simulink model "Model_Simscape_V3"  (R2023a)
settings: Solver=VariableStepAuto  StartTime=0.0  StopTime=10.0  RelTol=1e-3
model workspace (MAT data in the model file):
  Air_density = 1.29
  Body_Temperature = 37
  CtrlData_Max = 100
  CtrlData_Min = 0
  Detpress_to_Vavle : object (value not decoded)
  E_respriatory = 10
  ExpValve : object (value not decoded)
  FRC = 2
  Fan : object (value not decoded)
  FanHousing : object (value not decoded)
  Flow_Resistance_1 : object (value not decoded)
  Flow_Resistance_2 : object (value not decoded)
  Hard_Stop : Lower_bound (value not decoded)
  InspValve : object (value not decoded)
  L_to_m3 = 0.001
  Mask : object (value not decoded)
  OxyValve : object (value not decoded)
  OxygenSensor : object (value not decoded)
  Pa_to_cmH2O = 0.0101974428892
  Percent_to_Unit = 0.01
  Pipe_1 : object (value not decoded)
  Pipe_2 : object (value not decoded)
  Pipe_3 : object (value not decoded)
  R_respiratory = 2
  Reservoir : Cross_area (value not decoded)
  Trachea : object (value not decoded)
  Volume_Max = 0.9
  cmH2O_to_Pa = 98.0638
  cmH2O_to_kPa = 0.0981
  lung : object (value not decoded)
  percentage_to_rpm = 600
values from neighbouring files (symbols this model uses):
  MIN_TO_S = 60.0    [MVEPP_DataDict.sldd]
  TO_HUNDRED = 0.01    [MVEPP_DataDict.sldd]
  TO_MILLI = 1000.0    [MVEPP_DataDict.sldd]
symbols that are objects in the model workspace (value not decoded): FanHousing, Flow_Resistance_1, Flow_Resistance_2, InspValve, lung, OxygenSensor
libraries: fl_lib x83, nesl_utility x17, SimscapeFluids_lib x4, aerolibatmos2 x1
(part 3 of 4)

== system Model_Simscape_V3/Subsystem/DiverPressSensor ==
  Data Type Conversion5 : DataTypeConversion  OutDataTypeStr=single  SaturateOnIntegerOverflow=off  RndMeth=Floor
  PS-Simulink Converter : nesl_utility/PS-Simulink Converter  PhysicalDomain=network_engine_domain  SubClassName=ps_output  LeftPortType=input  RightPortType=output  PseudoPeriodic=off  Frequencies=[]  VectorFormat=inherit  Unit=Pa  AffineConversion=off
  Pressure & Temperature Sensor (G) : fl_lib/Gas/Sensors/Pressure & Temperature Sensor (G)  reference=foundation.enum.MeasurementReference.difference  pressure=true  pressure_spec=foundation.enum.PressureMeasementSpec.Absolute  temperature=false
      settings: InternalSimscapePortConfiguration="{\"Bottom\":[],\"Left\":[{\"id\":\"A\",\"label\":\"A\",\"type\":\"foundation.gas.gas\"}],\"Right\":[{\"id\":\"B\",\"label\":\"B\",\"type\":\"foundation.gas.gas\"},{\"id\":\"P\",\"label\":\"P\",\"type\":\"output\"}],\"Top\":[]}"
  Reservoir (G)1 : fl_lib/Gas/Elements/Reservoir (G)  pressure_spec=foundation.enum.pressure_spec.atmospheric  reservoir_pressure=0.101325 MPa  reservoir_temperature=293.15 K  area_A=Reservoir.Cross_area m^2
  Unit Conversion : UnitConversion
  A : PMIOPort  Side=Left
  Press : Outport  Unit=hPa
  wires:
  PS-Simulink Converter/1 -> Unit Conversion/1
  Unit Conversion/1 -> Data Type Conversion5/1
  Data Type Conversion5/1 -> Press/1
  connections:
  Reservoir (G)1/LConn1 -- Pressure & Temperature Sensor (G)/RConn1
  Pressure & Temperature Sensor (G)/LConn1 -- A/RConn1
  Pressure & Temperature Sensor (G)/RConn2 -- PS-Simulink Converter/LConn1

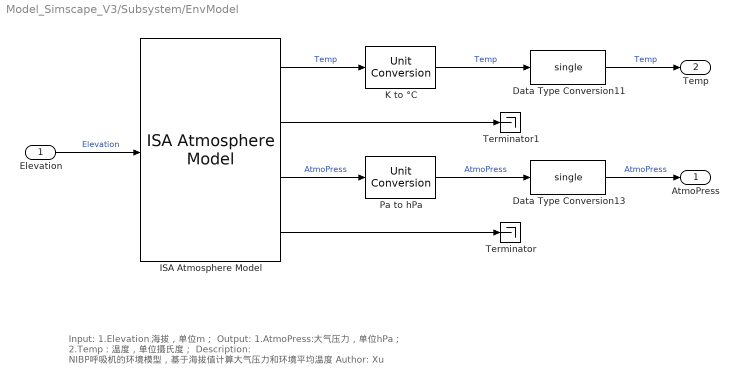
== system Model_Simscape_V3/Subsystem/EnvModel ==
  note: Input:
      | 	1.Elevation:海拔，单位m；
      | Output:
      | 	1.AtmoPress:大气压力，单位hPa；
      | 	2.Temp：温度，单位摄氏度；
      | Description:
      | 	NIBP呼吸机的环境模型，基于海拔值计算大气压力和环境平均温度
      | Author:
      | 	Xu
  Elevation : Inport  OutDataTypeStr=int16  Unit=m
  Data Type Conversion11 : DataTypeConversion  OutDataTypeStr=single  SaturateOnIntegerOverflow=off  RndMeth=Floor
  Data Type Conversion13 : DataTypeConversion  OutDataTypeStr=single  SaturateOnIntegerOverflow=off  RndMeth=Floor
  ISA Atmosphere Model : aerolibatmos2/ISA Atmosphere Model  custom=off  g=9.80665  gamma=1.4  R=287.0531  L=0.0065  h_trop=11000  h_strat=20000  rho0=1.225  P0=101325  T0=288.15  h0=0
  K to °C : UnitConversion  OutputType=Inherit: Inherit via back propagation
  Pa to hPa : UnitConversion  OutputType=Inherit: Inherit via back propagation
  Terminator : Terminator
  Terminator1 : Terminator
  AtmoPress : Outport  OutDataTypeStr=single  Unit=hPa
  Temp : Outport  Port=2  OutDataTypeStr=single  Unit=°C
  wires:
  Elevation/1 -> ISA Atmosphere Model/1  "Elevation"
  Pa to hPa/1 -> Data Type Conversion13/1  "AtmoPress"
  ISA Atmosphere Model/4 -> Terminator/1
  K to °C/1 -> Data Type Conversion11/1  "Temp"
  ISA Atmosphere Model/2 -> Terminator1/1
  ISA Atmosphere Model/3 -> Pa to hPa/1  "AtmoPress"
  ISA Atmosphere Model/1 -> K to °C/1  "Temp"
  Data Type Conversion11/1 -> Temp/1  "Temp"
  Data Type Conversion13/1 -> AtmoPress/1  "AtmoPress"

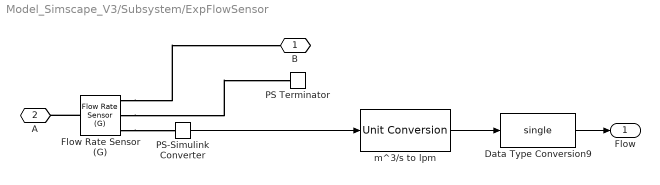
== system Model_Simscape_V3/Subsystem/ExpFlowSensor ==
  Data Type Conversion9 : DataTypeConversion  OutDataTypeStr=single  SaturateOnIntegerOverflow=off  RndMeth=Floor
  Flow Rate Sensor (G) : fl_lib/Gas/Sensors/Flow Rate Sensor (G)  mass_flow_measure=true  volumetric_flow_measure=true  volumetric_flow_conditions=foundation.enum.volumetric_flow_conditions.actual  p_std=0.101325 MPa  T_std=20 degC  energy_flow_measure=false
      settings: InternalSimscapePortConfiguration="{\"Bottom\":[],\"Left\":[{\"id\":\"A\",\"label\":\"A\",\"type\":\"foundation.gas.gas\"}],\"Right\":[{\"id\":\"B\",\"label\":\"B\",\"type\":\"foundation.gas.gas\"},{\"id\":\"M\",\"label\":\"M\",\"type\":\"output\"},{\"id\":\"V\",\"label\":\"V\",\"type\":\"output\"}],\"Top\":[]}"
  PS Terminator : fl_lib/Physical Signals/Sinks/PS Terminator
  PS-Simulink Converter : nesl_utility/PS-Simulink Converter  PhysicalDomain=network_engine_domain  SubClassName=ps_output  LeftPortType=input  RightPortType=output  PseudoPeriodic=off  Frequencies=[]  VectorFormat=inherit  Unit=m^3/s  AffineConversion=off
  m^3/s to lpm : UnitConversion
  B : PMIOPort  Side=Left
  A : PMIOPort  Port=2  Side=Right
  Flow : Outport  Unit=lpm
  wires:
  PS-Simulink Converter/1 -> m^3/s to lpm/1
  m^3/s to lpm/1 -> Data Type Conversion9/1
  Data Type Conversion9/1 -> Flow/1
  connections:
  Flow Rate Sensor (G)/RConn1 -- B/RConn1
  Flow Rate Sensor (G)/LConn1 -- A/RConn1
  Flow Rate Sensor (G)/RConn2 -- PS Terminator/LConn1
  Flow Rate Sensor (G)/RConn3 -- PS-Simulink Converter/LConn1

== system Model_Simscape_V3/Subsystem/ExpPawSensor ==
  Data Type Conversion8 : DataTypeConversion  OutDataTypeStr=single  SaturateOnIntegerOverflow=off  RndMeth=Floor
  PS-Simulink Converter : nesl_utility/PS-Simulink Converter  PhysicalDomain=network_engine_domain  SubClassName=ps_output  LeftPortType=input  RightPortType=output  PseudoPeriodic=off  Frequencies=[]  VectorFormat=inherit  Unit=inherit  AffineConversion=off
  Pressure & Temperature Sensor (G) : fl_lib/Gas/Sensors/Pressure & Temperature Sensor (G)  reference=foundation.enum.MeasurementReference.difference  pressure=true  pressure_spec=foundation.enum.PressureMeasementSpec.Absolute  temperature=false
      settings: InternalSimscapePortConfiguration="{\"Bottom\":[],\"Left\":[{\"id\":\"A\",\"label\":\"A\",\"type\":\"foundation.gas.gas\"}],\"Right\":[{\"id\":\"B\",\"label\":\"B\",\"type\":\"foundation.gas.gas\"},{\"id\":\"P\",\"label\":\"P\",\"type\":\"output\"}],\"Top\":[]}"
  Reservoir (G)1 : fl_lib/Gas/Elements/Reservoir (G)  pressure_spec=foundation.enum.pressure_spec.atmospheric  reservoir_pressure=0.101325 MPa  reservoir_temperature=293.15 K  area_A=Reservoir.Cross_area m^2
  Unit Conversion : UnitConversion
  A : PMIOPort  Side=Left
  Press : Outport  Unit=hPa
  wires:
  PS-Simulink Converter/1 -> Unit Conversion/1
  Unit Conversion/1 -> Data Type Conversion8/1
  Data Type Conversion8/1 -> Press/1
  connections:
  PS-Simulink Converter/LConn1 -- Pressure & Temperature Sensor (G)/RConn2
  Reservoir (G)1/LConn1 -- Pressure & Temperature Sensor (G)/RConn1
  Pressure & Temperature Sensor (G)/LConn1 -- A/RConn1

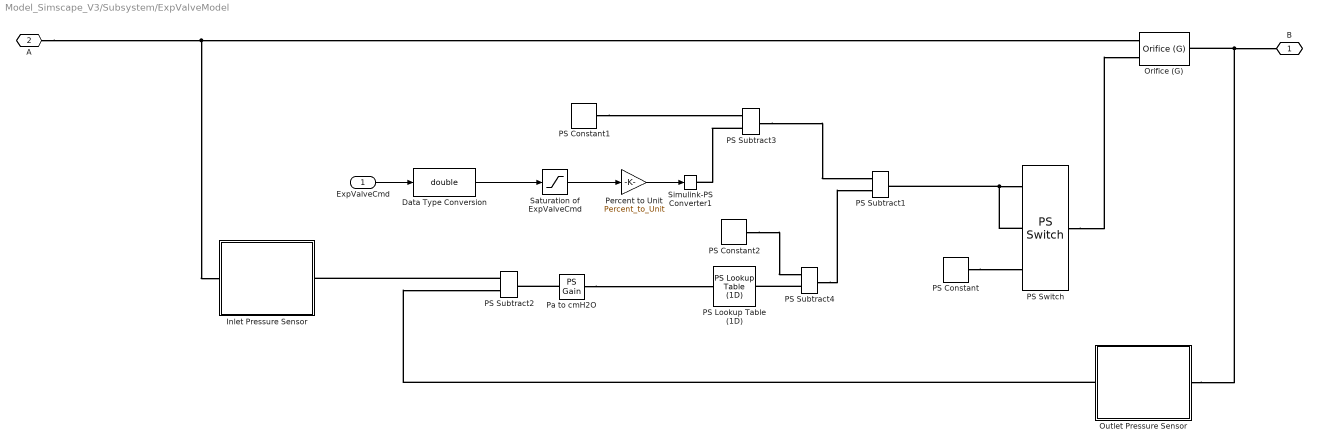
== system Model_Simscape_V3/Subsystem/ExpValveModel ==
  ExpValveCmd : Inport
  " Inlet Pressure Sensor" : Subsystem
  " Outlet Pressure Sensor" : Subsystem
  Data Type Conversion : DataTypeConversion  OutDataTypeStr=double  SaturateOnIntegerOverflow=off  RndMeth=Floor
  Orifice (G) : SimscapeFluids_lib/Gas/Valves & Orifices/Orifice (G)  orifice_type=foundation.enum.constant_variable.variable  orifice_parameterization=fluids.gas.valves_orifices.enum.OrificeParameterization.Cv  opening_characteristic=fluids.gas.valves_orifices.enum.OpeningCharacteristics.Tabulated  Cv_constant=4  Cv_max=4  L_Cv_TLU=ExpValve.opening_vector  Cv_TLU=ExpValve.Cv_vector  xT_Cv=0.7  Kv_constant=3.6  Kv_max=3.6  L_Kv_TLU=0 : 0.2 : 1  Kv_TLU=[1e-06, .72, 1.44, 2.16, 2.88, 3.6]  xT_Kv=0.7  C_constant=12 l/(bar*s)  B_crit_constant=0.3  C_max=12 l/(bar*s)  B_crit_linear=0.3  L_C_TLU=0 : 0.2 : 1  C_TLU=[1e-05, 2.4, 4.8, 7.2, 9.6, 12] l/(bar*s)  B_crit_TLU=0.3 * ones(1, 6)  m=0.5  T_ref_C=293.15 K  rho_ref_C=1.185 kg/m^3  orifice_area_constant=1e-4 m^2  orifice_area_max=1e-4 m^2  L_orifice_area_TLU=0 : 0.2 : 1  orifice_area_TLU=[1e-10, 2e-05, 4e-05, 6e-05, 8e-05, .0001] m^2  Cd=0.64  leakage_fraction=1e-6  smoothing_factor=0.01  B_lam=0.999  area=ExpValve.Cross_Area m^2
      settings: InternalSimscapePortConfiguration="{\"Bottom\":[],\"Left\":[{\"id\":\"A\",\"label\":\"A\",\"type\":\"foundation.gas.gas\"},{\"id\":\"L\",\"label\":\"L\",\"type\":\"input\"}],\"Right\":[{\"id\":\"B\",\"label\":\"B\",\"type\":\"foundation.gas.gas\"}],\"Top\":[]}"
  PS Constant : fl_lib/Physical Signals/Sources/PS Constant  constant=ExpValve.zerovalue
  PS Constant1 : fl_lib/Physical Signals/Sources/PS Constant  constant=ExpValve.fullValue
  PS Constant2 : fl_lib/Physical Signals/Sources/PS Constant  constant=ExpValve.fullValue
  PS Lookup Table (1D) : fl_lib/Physical Signals/Lookup Tables/PS Lookup Table (1D)  x=Detpress_to_Vavle.detpress  f=Detpress_to_Vavle.vavle  interp_method=simscape.enum.interpolation.linear  extrap_method=simscape.enum.extrapolation.nearest
  PS Subtract{1..4} (4 alike) : fl_lib/Physical Signals/Functions/PS Subtract
  PS Switch : fl_lib/Physical Signals/Nonlinear Operators/PS Switch  Threshold=0.001
      settings: InternalSimscapePortConfiguration="{\"Bottom\":[],\"Left\":[{\"id\":\"I1\",\"label\":\"\",\"type\":\"input\"},{\"id\":\"I2\",\"label\":\"\",\"type\":\"input\"},{\"id\":\"I3\",\"label\":\"\",\"type\":\"input\"}],\"Right\":[{\"id\":\"O\",\"label\":\"\",\"type\":\"output\"}],\"Top\":[]}"
  Pa to cmH2O : fl_lib/Physical Signals/Functions/PS Gain  gain=Pa_to_cmH2O 1/Pa
  Percent to Unit : Gain  Gain=Percent_to_Unit
  Saturation of ExpValveCmd : Saturate  UpperLimit=CtrlData_Max  LowerLimit=CtrlData_Min
  Simulink-PS Converter1 : nesl_utility/Simulink-PS Converter  PhysicalDomain=network_engine_domain  SubClassName=ps_input  LeftPortType=input  RightPortType=output  PseudoPeriodic=off  Frequencies=[]  NoiseDistribution=none  NoiseParameters=[]  Unit=1  AffineConversion=off  FilteringAndDerivatives=provide  SimscapeFilterOrder=1  InputFilterTimeConstant=0.001  UdotUserProvided=0
  B : PMIOPort  Side=Left
  A : PMIOPort  Port=2  Side=Right
  wires:
  Percent to Unit/1 -> Simulink-PS Converter1/1
  ExpValveCmd/1 -> Data Type Conversion/1
  Saturation of ExpValveCmd/1 -> Percent to Unit/1
  Data Type Conversion/1 -> Saturation of ExpValveCmd/1
  connections:
  " Outlet Pressure Sensor"/RConn1 -- Orifice (G)/RConn1 -- B/RConn1
  PS Subtract2/LConn1 -- " Inlet Pressure Sensor"/RConn1
  PS Constant/RConn1 -- PS Switch/LConn3
  PS Switch/LConn2 -- PS Subtract1/RConn1 -- PS Switch/LConn1
  " Outlet Pressure Sensor"/LConn1 -- PS Subtract2/LConn2
  A/RConn1 -- Orifice (G)/LConn1 -- " Inlet Pressure Sensor"/LConn1
  PS Switch/RConn1 -- Orifice (G)/LConn2
  Pa to cmH2O/LConn1 -- PS Subtract2/RConn1
  Pa to cmH2O/RConn1 -- PS Lookup Table (1D)/LConn1
  PS Subtract3/LConn2 -- Simulink-PS Converter1/RConn1
  PS Subtract3/RConn1 -- PS Subtract1/LConn1
  PS Constant1/RConn1 -- PS Subtract3/LConn1
  PS Subtract4/LConn2 -- PS Lookup Table (1D)/RConn1
  PS Constant2/RConn1 -- PS Subtract4/LConn1
  PS Subtract4/RConn1 -- PS Subtract1/LConn2

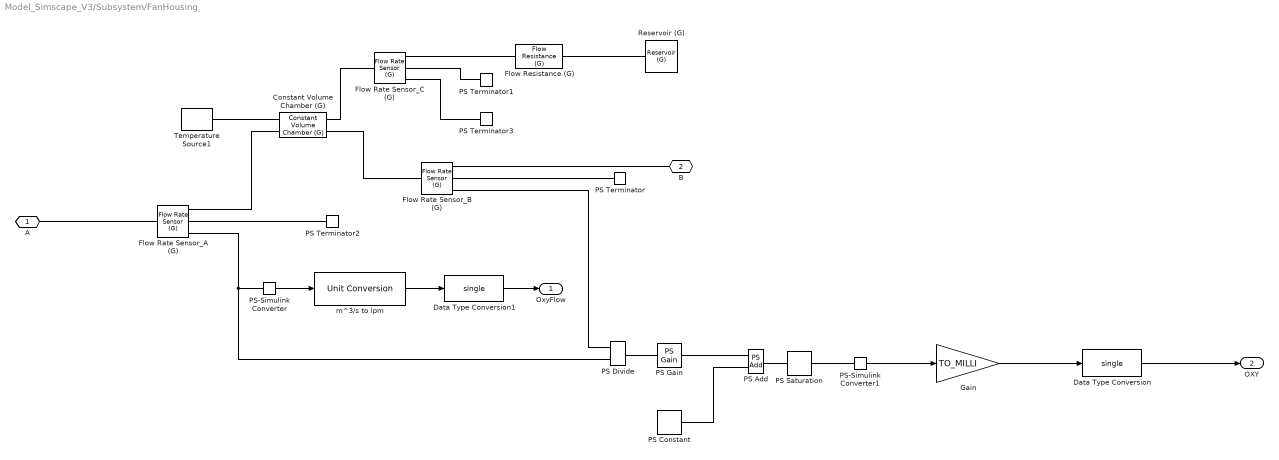
== system Model_Simscape_V3/Subsystem/FanHousing ==
  Constant Volume Chamber (G) : fl_lib/Gas/Elements/Constant Volume Chamber (G)  volume=FanHousing.Chamber_volume m^3  num_ports=foundation.enum.num_ports.three  area_A=FanHousing.A_area m^2  area_B=FanHousing.B_area m^2  area_C=FanHousing.C_area m^2  area_D=0.01 m^2  p_I_specify=off  p_I_priority=High  p_I=0.101325 MPa  p_I_nominal_specify=off  p_I_nominal_unit=MPa  p_I_nominal_value=1  T_I_specify=off  T_I_priority=High  T_I=293.15 K  T_I_nominal_specify=off  T_I_nominal_unit=K  T_I_nominal_value=1  rho_I_specify=off  rho_I_priority=None  rho_I=1.2 kg/m^3  rho_I_nominal_specify=off  rho_I_nominal_unit=kg/m^3  rho_I_nominal_value=1
      settings: InternalSimscapePortConfiguration="{\"Bottom\":[],\"Left\":[{\"id\":\"A\",\"label\":\"A\",\"type\":\"foundation.gas.gas\"},{\"id\":\"H\",\"label\":\"H\",\"type\":\"foundation.thermal.thermal\"}],\"Right\":[{\"id\":\"B\",\"label\":\"B\",\"type\":\"foundation.gas.gas\"},{\"id\":\"C\",\"label\":\"C\",\"type\":\"foundation.gas.gas\"}],\"Top\":[]}"
  Data Type Conversion : DataTypeConversion  OutDataTypeStr=single  SaturateOnIntegerOverflow=off  RndMeth=Floor
  Data Type Conversion1 : DataTypeConversion  OutDataTypeStr=single  SaturateOnIntegerOverflow=off  RndMeth=Floor
  Flow Rate Sensor_A (G) : fl_lib/Gas/Sensors/Flow Rate Sensor (G)  mass_flow_measure=true  volumetric_flow_measure=true  volumetric_flow_conditions=foundation.enum.volumetric_flow_conditions.actual  p_std=0.101325 MPa  T_std=20 degC  energy_flow_measure=false
      settings: InternalSimscapePortConfiguration="{\"Bottom\":[],\"Left\":[{\"id\":\"A\",\"label\":\"A\",\"type\":\"foundation.gas.gas\"}],\"Right\":[{\"id\":\"B\",\"label\":\"B\",\"type\":\"foundation.gas.gas\"},{\"id\":\"M\",\"label\":\"M\",\"type\":\"output\"},{\"id\":\"V\",\"label\":\"V\",\"type\":\"output\"}],\"Top\":[]}"
  Flow Rate Sensor_B (G) : fl_lib/Gas/Sensors/Flow Rate Sensor (G)  mass_flow_measure=true  volumetric_flow_measure=true  volumetric_flow_conditions=foundation.enum.volumetric_flow_conditions.actual  p_std=0.101325 MPa  T_std=20 degC  energy_flow_measure=false
      settings: InternalSimscapePortConfiguration="{\"Bottom\":[],\"Left\":[{\"id\":\"A\",\"label\":\"A\",\"type\":\"foundation.gas.gas\"}],\"Right\":[{\"id\":\"B\",\"label\":\"B\",\"type\":\"foundation.gas.gas\"},{\"id\":\"M\",\"label\":\"M\",\"type\":\"output\"},{\"id\":\"V\",\"label\":\"V\",\"type\":\"output\"}],\"Top\":[]}"
  Flow Rate Sensor_C (G) : fl_lib/Gas/Sensors/Flow Rate Sensor (G)  mass_flow_measure=true  volumetric_flow_measure=true  volumetric_flow_conditions=foundation.enum.volumetric_flow_conditions.actual  p_std=0.101325 MPa  T_std=20 degC  energy_flow_measure=false
      settings: InternalSimscapePortConfiguration="{\"Bottom\":[],\"Left\":[{\"id\":\"A\",\"label\":\"A\",\"type\":\"foundation.gas.gas\"}],\"Right\":[{\"id\":\"B\",\"label\":\"B\",\"type\":\"foundation.gas.gas\"},{\"id\":\"M\",\"label\":\"M\",\"type\":\"output\"},{\"id\":\"V\",\"label\":\"V\",\"type\":\"output\"}],\"Top\":[]}"
  Flow Resistance (G) : fl_lib/Gas/Elements/Flow Resistance (G)  delta_p_nominal=FanHousing.pressure_drop*cmH2O_to_kPa kPa  mdot_nominal=FanHousing.flow_rate*L_to_m3*Air_density kg/s  rho_nominal=0 kg/m^3  area="FanHousing.Crosss_Area  m^2"  laminar_fraction=1e-3
      settings: InternalSimscapePortConfiguration="{\"Bottom\":[],\"Left\":[{\"id\":\"A\",\"label\":\"A\",\"type\":\"foundation.gas.gas\"}],\"Right\":[{\"id\":\"B\",\"label\":\"B\",\"type\":\"foundation.gas.gas\"}],\"Top\":[]}"
  Gain : Gain  Gain=TO_MILLI
  PS Add : fl_lib/Physical Signals/Functions/PS Add
  PS Constant : fl_lib/Physical Signals/Sources/PS Constant  constant=OxygenSensor.Air_oxygen_concentration
  PS Divide : fl_lib/Physical Signals/Functions/PS Divide
  PS Gain : fl_lib/Physical Signals/Functions/PS Gain  gain=OxygenSensor.K
  PS Saturation : fl_lib/Physical Signals/Nonlinear Operators/PS Saturation  upper_limit=1  lower_limit=0
  PS Terminator{,1..3} (4 alike) : fl_lib/Physical Signals/Sinks/PS Terminator
  PS-Simulink Converter : nesl_utility/PS-Simulink Converter  PhysicalDomain=network_engine_domain  SubClassName=ps_output  LeftPortType=input  RightPortType=output  PseudoPeriodic=off  Frequencies=[]  VectorFormat=inherit  Unit=m^3/s  AffineConversion=off
  PS-Simulink Converter1 : nesl_utility/PS-Simulink Converter  PhysicalDomain=network_engine_domain  SubClassName=ps_output  LeftPortType=input  RightPortType=output  PseudoPeriodic=off  Frequencies=[]  VectorFormat=inherit  Unit=1  AffineConversion=off
  Reservoir (G) : fl_lib/Gas/Elements/Reservoir (G)  pressure_spec=foundation.enum.pressure_spec.atmospheric  reservoir_pressure=0.101325 MPa  reservoir_temperature=293.15 K  area_A=0.01 m^2
  Temperature Source1 : fl_lib/Thermal/Thermal Sources/Temperature Source  temperature=293.15 K
  m^3/s to lpm : UnitConversion
  A : PMIOPort  Side=Left
  B : PMIOPort  Port=2  Side=Right
  OxyFlow : Outport  Unit=lpm
  OXY : Outport  Port=2  Unit=m
  wires:
  PS-Simulink Converter/1 -> m^3/s to lpm/1
  m^3/s to lpm/1 -> Data Type Conversion1/1
  PS-Simulink Converter1/1 -> Gain/1
  Gain/1 -> Data Type Conversion/1
  Data Type Conversion/1 -> OXY/1
  Data Type Conversion1/1 -> OxyFlow/1
  connections:
  Flow Rate Sensor_C (G)/RConn2 -- PS Terminator1/LConn1
  PS Terminator2/LConn1 -- Flow Rate Sensor_A (G)/RConn2
  Flow Rate Sensor_C (G)/RConn3 -- PS Terminator3/LConn1
  PS Terminator/LConn1 -- Flow Rate Sensor_B (G)/RConn2
  Flow Rate Sensor_C (G)/LConn1 -- Constant Volume Chamber (G)/RConn2
  Constant Volume Chamber (G)/RConn1 -- Flow Rate Sensor_B (G)/LConn1
  Flow Resistance (G)/LConn1 -- Flow Rate Sensor_C (G)/RConn1
  Reservoir (G)/LConn1 -- Flow Resistance (G)/RConn1
  Flow Rate Sensor_B (G)/RConn1 -- B/RConn1
  Constant Volume Chamber (G)/LConn1 -- Flow Rate Sensor_A (G)/RConn1
  Temperature Source1/LConn1 -- Constant Volume Chamber (G)/LConn2
  A/RConn1 -- Flow Rate Sensor_A (G)/LConn1
  Flow Rate Sensor_B (G)/RConn3 -- PS Divide/LConn2
  Flow Rate Sensor_A (G)/RConn3 -- PS Divide/LConn1 -- PS-Simulink Converter/LConn1
  PS Gain/LConn1 -- PS Divide/RConn1
  PS Constant/RConn1 -- PS Add/LConn2
  PS Gain/RConn1 -- PS Add/LConn1
  PS Saturation/LConn1 -- PS Add/RConn1
  PS-Simulink Converter1/LConn1 -- PS Saturation/RConn1

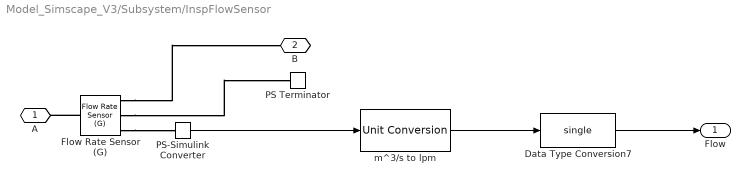
== system Model_Simscape_V3/Subsystem/InspFlowSensor  ==
  Data Type Conversion7 : DataTypeConversion  OutDataTypeStr=single  SaturateOnIntegerOverflow=off  RndMeth=Floor
  Flow Rate Sensor (G) : fl_lib/Gas/Sensors/Flow Rate Sensor (G)  mass_flow_measure=true  volumetric_flow_measure=true  volumetric_flow_conditions=foundation.enum.volumetric_flow_conditions.actual  p_std=0.101325 MPa  T_std=20 degC  energy_flow_measure=false
      settings: InternalSimscapePortConfiguration="{\"Bottom\":[],\"Left\":[{\"id\":\"A\",\"label\":\"A\",\"type\":\"foundation.gas.gas\"}],\"Right\":[{\"id\":\"B\",\"label\":\"B\",\"type\":\"foundation.gas.gas\"},{\"id\":\"M\",\"label\":\"M\",\"type\":\"output\"},{\"id\":\"V\",\"label\":\"V\",\"type\":\"output\"}],\"Top\":[]}"
  PS Terminator : fl_lib/Physical Signals/Sinks/PS Terminator
  PS-Simulink Converter : nesl_utility/PS-Simulink Converter  PhysicalDomain=network_engine_domain  SubClassName=ps_output  LeftPortType=input  RightPortType=output  PseudoPeriodic=off  Frequencies=[]  VectorFormat=inherit  Unit=m^3/s  AffineConversion=off
  m^3/s to lpm : UnitConversion
  A : PMIOPort  Side=Left
  B : PMIOPort  Port=2  Side=Right
  Flow : Outport  Unit=lpm
  wires:
  PS-Simulink Converter/1 -> m^3/s to lpm/1
  m^3/s to lpm/1 -> Data Type Conversion7/1
  Data Type Conversion7/1 -> Flow/1
  connections:
  Flow Rate Sensor (G)/RConn1 -- B/RConn1
  Flow Rate Sensor (G)/LConn1 -- A/RConn1
  Flow Rate Sensor (G)/RConn2 -- PS Terminator/LConn1
  Flow Rate Sensor (G)/RConn3 -- PS-Simulink Converter/LConn1

== system Model_Simscape_V3/Subsystem/InspPawSensor ==
  Data Type Conversion6 : DataTypeConversion  OutDataTypeStr=single  SaturateOnIntegerOverflow=off  RndMeth=Floor
  PS-Simulink Converter : nesl_utility/PS-Simulink Converter  PhysicalDomain=network_engine_domain  SubClassName=ps_output  LeftPortType=input  RightPortType=output  PseudoPeriodic=off  Frequencies=[]  VectorFormat=inherit  Unit=inherit  AffineConversion=off
  Pressure & Temperature Sensor (G) : fl_lib/Gas/Sensors/Pressure & Temperature Sensor (G)  reference=foundation.enum.MeasurementReference.difference  pressure=true  pressure_spec=foundation.enum.PressureMeasementSpec.Absolute  temperature=false
      settings: InternalSimscapePortConfiguration="{\"Bottom\":[],\"Left\":[{\"id\":\"A\",\"label\":\"A\",\"type\":\"foundation.gas.gas\"}],\"Right\":[{\"id\":\"B\",\"label\":\"B\",\"type\":\"foundation.gas.gas\"},{\"id\":\"P\",\"label\":\"P\",\"type\":\"output\"}],\"Top\":[]}"
  Reservoir (G)1 : fl_lib/Gas/Elements/Reservoir (G)  pressure_spec=foundation.enum.pressure_spec.atmospheric  reservoir_pressure=0.101325 MPa  reservoir_temperature=293.15 K  area_A=Reservoir.Cross_area m^2
  Unit Conversion : UnitConversion
  A : PMIOPort  Side=Left
  Press : Outport  Unit=hPa
  wires:
  PS-Simulink Converter/1 -> Unit Conversion/1
  Unit Conversion/1 -> Data Type Conversion6/1
  Data Type Conversion6/1 -> Press/1
  connections:
  Pressure & Temperature Sensor (G)/LConn1 -- A/RConn1
  Reservoir (G)1/LConn1 -- Pressure & Temperature Sensor (G)/RConn1
  PS-Simulink Converter/LConn1 -- Pressure & Temperature Sensor (G)/RConn2

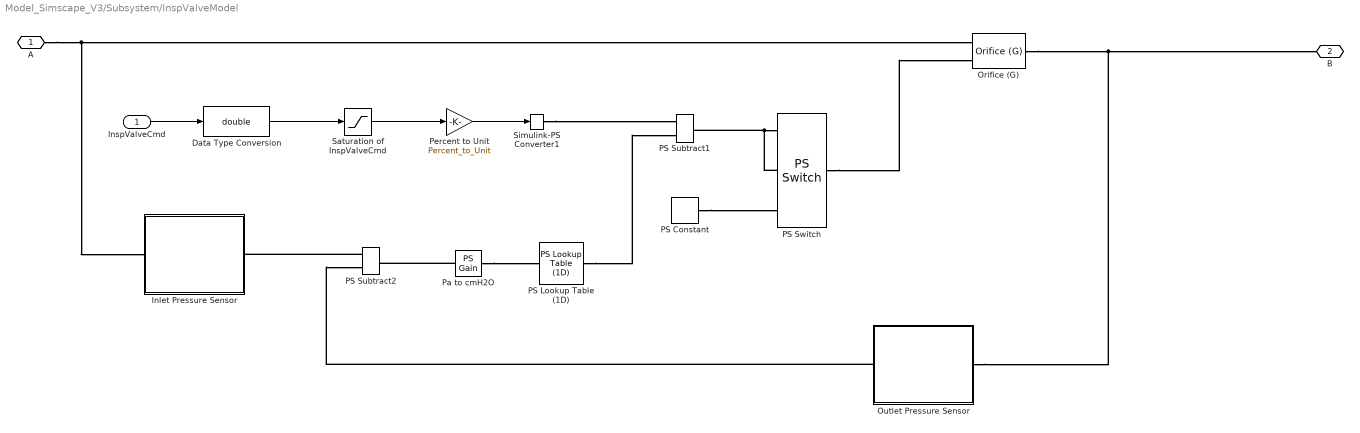
== system Model_Simscape_V3/Subsystem/InspValveModel ==
  InspValveCmd : Inport
  " Inlet Pressure Sensor" : Subsystem
  " Outlet Pressure Sensor" : Subsystem
  Data Type Conversion : DataTypeConversion  OutDataTypeStr=double  SaturateOnIntegerOverflow=off  RndMeth=Floor
  Orifice (G) : SimscapeFluids_lib/Gas/Valves & Orifices/Orifice (G)  orifice_type=foundation.enum.constant_variable.variable  orifice_parameterization=fluids.gas.valves_orifices.enum.OrificeParameterization.Cv  opening_characteristic=fluids.gas.valves_orifices.enum.OpeningCharacteristics.Tabulated  Cv_constant=4  Cv_max=4  L_Cv_TLU=InspValve.opening_vector  Cv_TLU=InspValve.Cv_vector  xT_Cv=0.7  Kv_constant=3.6  Kv_max=3.6  L_Kv_TLU=0 : 0.2 : 1  Kv_TLU=[1e-06, .72, 1.44, 2.16, 2.88, 3.6]  xT_Kv=0.7  C_constant=12 l/(bar*s)  B_crit_constant=0.3  C_max=12 l/(bar*s)  B_crit_linear=0.3  L_C_TLU=0 : 0.2 : 1  C_TLU=[1e-05, 2.4, 4.8, 7.2, 9.6, 12] l/(bar*s)  B_crit_TLU=0.3 * ones(1, 6)  m=0.5  T_ref_C=293.15 K  rho_ref_C=1.185 kg/m^3  orifice_area_constant=1e-4 m^2  orifice_area_max=1e-4 m^2  L_orifice_area_TLU=0 : 0.2 : 1  orifice_area_TLU=[1e-10, 2e-05, 4e-05, 6e-05, 8e-05, .0001] m^2  Cd=0.64  leakage_fraction=1e-6  smoothing_factor=0.01  B_lam=0.999  area=InspValve.Cross_Area m^2
      settings: InternalSimscapePortConfiguration="{\"Bottom\":[],\"Left\":[{\"id\":\"A\",\"label\":\"A\",\"type\":\"foundation.gas.gas\"},{\"id\":\"L\",\"label\":\"L\",\"type\":\"input\"}],\"Right\":[{\"id\":\"B\",\"label\":\"B\",\"type\":\"foundation.gas.gas\"}],\"Top\":[]}"
  PS Constant : fl_lib/Physical Signals/Sources/PS Constant  constant=InspValve.zerovalue
  PS Lookup Table (1D) : fl_lib/Physical Signals/Lookup Tables/PS Lookup Table (1D)  x=Detpress_to_Vavle.detpress  f=Detpress_to_Vavle.vavle  interp_method=simscape.enum.interpolation.linear  extrap_method=simscape.enum.extrapolation.nearest
  PS Subtract1 : fl_lib/Physical Signals/Functions/PS Subtract
  PS Subtract2 : fl_lib/Physical Signals/Functions/PS Subtract
  PS Switch : fl_lib/Physical Signals/Nonlinear Operators/PS Switch  Threshold=InspValve.zerovalue
      settings: InternalSimscapePortConfiguration="{\"Bottom\":[],\"Left\":[{\"id\":\"I1\",\"label\":\"\",\"type\":\"input\"},{\"id\":\"I2\",\"label\":\"\",\"type\":\"input\"},{\"id\":\"I3\",\"label\":\"\",\"type\":\"input\"}],\"Right\":[{\"id\":\"O\",\"label\":\"\",\"type\":\"output\"}],\"Top\":[]}"
  Pa to cmH2O : fl_lib/Physical Signals/Functions/PS Gain  gain=Pa_to_cmH2O 1/Pa
  Percent to Unit : Gain  Gain=Percent_to_Unit
  Saturation of InspValveCmd : Saturate  UpperLimit=CtrlData_Max  LowerLimit=CtrlData_Min
  Simulink-PS Converter1 : nesl_utility/Simulink-PS Converter  PhysicalDomain=network_engine_domain  SubClassName=ps_input  LeftPortType=input  RightPortType=output  PseudoPeriodic=off  Frequencies=[]  NoiseDistribution=none  NoiseParameters=[]  Unit=1  AffineConversion=off  FilteringAndDerivatives=provide  SimscapeFilterOrder=1  InputFilterTimeConstant=0.001  UdotUserProvided=0
  A : PMIOPort  Side=Left
  B : PMIOPort  Port=2  Side=Right
  wires:
  InspValveCmd/1 -> Data Type Conversion/1
  Percent to Unit/1 -> Simulink-PS Converter1/1
  Saturation of InspValveCmd/1 -> Percent to Unit/1
  Data Type Conversion/1 -> Saturation of InspValveCmd/1
  connections:
  Orifice (G)/RConn1 -- " Outlet Pressure Sensor"/RConn1 -- B/RConn1
  PS Subtract2/LConn1 -- " Inlet Pressure Sensor"/RConn1
  PS Constant/RConn1 -- PS Switch/LConn3
  PS Switch/LConn2 -- PS Subtract1/RConn1 -- PS Switch/LConn1
  PS Lookup Table (1D)/RConn1 -- PS Subtract1/LConn2
  " Outlet Pressure Sensor"/LConn1 -- PS Subtract2/LConn2
  A/RConn1 -- Orifice (G)/LConn1 -- " Inlet Pressure Sensor"/LConn1
  Simulink-PS Converter1/RConn1 -- PS Subtract1/LConn1
  PS Switch/RConn1 -- Orifice (G)/LConn2
  Pa to cmH2O/LConn1 -- PS Subtract2/RConn1
  Pa to cmH2O/RConn1 -- PS Lookup Table (1D)/LConn1

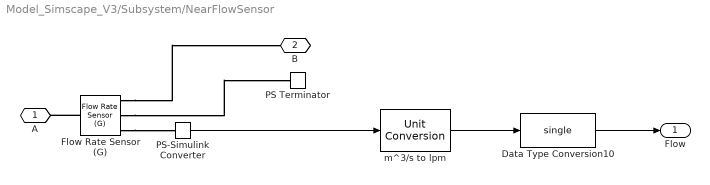
== system Model_Simscape_V3/Subsystem/NearFlowSensor  ==
  Data Type Conversion10 : DataTypeConversion  OutDataTypeStr=single  SaturateOnIntegerOverflow=off  RndMeth=Floor
  Flow Rate Sensor (G) : fl_lib/Gas/Sensors/Flow Rate Sensor (G)  mass_flow_measure=true  volumetric_flow_measure=true  volumetric_flow_conditions=foundation.enum.volumetric_flow_conditions.actual  p_std=0.101325 MPa  T_std=20 degC  energy_flow_measure=false
      settings: InternalSimscapePortConfiguration="{\"Bottom\":[],\"Left\":[{\"id\":\"A\",\"label\":\"A\",\"type\":\"foundation.gas.gas\"}],\"Right\":[{\"id\":\"B\",\"label\":\"B\",\"type\":\"foundation.gas.gas\"},{\"id\":\"M\",\"label\":\"M\",\"type\":\"output\"},{\"id\":\"V\",\"label\":\"V\",\"type\":\"output\"}],\"Top\":[]}"
  PS Terminator : fl_lib/Physical Signals/Sinks/PS Terminator
  PS-Simulink Converter : nesl_utility/PS-Simulink Converter  PhysicalDomain=network_engine_domain  SubClassName=ps_output  LeftPortType=input  RightPortType=output  PseudoPeriodic=off  Frequencies=[]  VectorFormat=inherit  Unit=m^3/s  AffineConversion=off
  m^3/s to lpm : UnitConversion
  A : PMIOPort  Side=Left
  B : PMIOPort  Port=2  Side=Right
  Flow : Outport  Unit=lpm
  wires:
  m^3/s to lpm/1 -> Data Type Conversion10/1
  PS-Simulink Converter/1 -> m^3/s to lpm/1
  Data Type Conversion10/1 -> Flow/1
  connections:
  Flow Rate Sensor (G)/RConn3 -- PS-Simulink Converter/LConn1
  Flow Rate Sensor (G)/RConn2 -- PS Terminator/LConn1
  Flow Rate Sensor (G)/LConn1 -- A/RConn1
  Flow Rate Sensor (G)/RConn1 -- B/RConn1

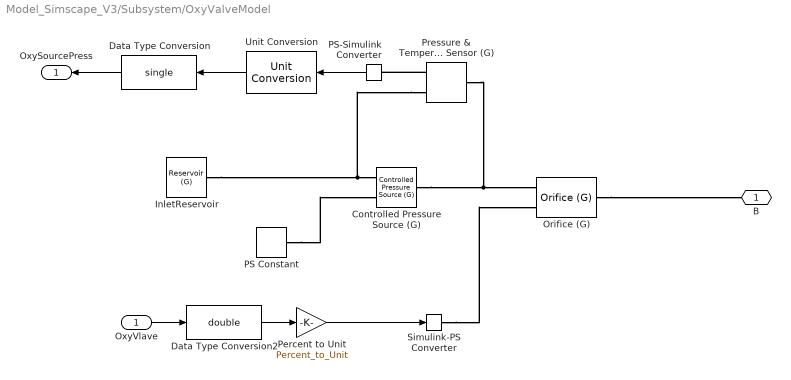
== system Model_Simscape_V3/Subsystem/OxyValveModel ==
  OxyVlave : Inport
  Controlled Pressure Source (G) : fl_lib/Gas/Sources/Controlled Pressure Source (G)  power_spec=foundation.enum.power_spec.isentropic  area_A=0.01 m^2  area_B=0.01 m^2
      settings: InternalSimscapePortConfiguration="{\"Bottom\":[],\"Left\":[{\"id\":\"A\",\"label\":\"A\",\"type\":\"foundation.gas.gas\"},{\"id\":\"P\",\"label\":\"P\",\"type\":\"input\"}],\"Right\":[{\"id\":\"B\",\"label\":\"B\",\"type\":\"foundation.gas.gas\"}],\"Top\":[]}"
  Data Type Conversion : DataTypeConversion  OutDataTypeStr=single  SaturateOnIntegerOverflow=off  RndMeth=Floor
  Data Type Conversion2 : DataTypeConversion  OutDataTypeStr=double  SaturateOnIntegerOverflow=off  RndMeth=Floor
  InletReservoir : fl_lib/Gas/Elements/Reservoir (G)  pressure_spec=foundation.enum.pressure_spec.atmospheric  reservoir_pressure=0.101325 MPa  reservoir_temperature=293.15 K  area_A=Reservoir.Cross_area m^2
  Orifice (G) : SimscapeFluids_lib/Gas/Valves & Orifices/Orifice (G)  orifice_type=foundation.enum.constant_variable.variable  orifice_parameterization=fluids.gas.valves_orifices.enum.OrificeParameterization.Cv  opening_characteristic=fluids.gas.valves_orifices.enum.OpeningCharacteristics.Tabulated  Cv_constant=4  Cv_max=4  L_Cv_TLU=OxyValve.opening_vector  Cv_TLU=OxyValve.Cv_vector  xT_Cv=0.7  Kv_constant=3.6  Kv_max=3.6  L_Kv_TLU=0 : 0.2 : 1  Kv_TLU=[1e-06, .72, 1.44, 2.16, 2.88, 3.6]  xT_Kv=0.7  C_constant=12 l/(bar*s)  B_crit_constant=0.3  C_max=12 l/(bar*s)  B_crit_linear=0.3  L_C_TLU=0 : 0.2 : 1  C_TLU=[1e-05, 2.4, 4.8, 7.2, 9.6, 12] l/(bar*s)  B_crit_TLU=0.3 * ones(1, 6)  m=0.5  T_ref_C=293.15 K  rho_ref_C=1.185 kg/m^3  orifice_area_constant=1e-4 m^2  orifice_area_max=1e-4 m^2  L_orifice_area_TLU=0 : 0.2 : 1  orifice_area_TLU=[1e-10, 2e-05, 4e-05, 6e-05, 8e-05, .0001] m^2  Cd=0.64  leakage_fraction=1e-6  smoothing_factor=0.01  B_lam=0.999  area=OxyValve.Cross_Area m^2
      settings: InternalSimscapePortConfiguration="{\"Bottom\":[],\"Left\":[{\"id\":\"A\",\"label\":\"A\",\"type\":\"foundation.gas.gas\"},{\"id\":\"L\",\"label\":\"L\",\"type\":\"input\"}],\"Right\":[{\"id\":\"B\",\"label\":\"B\",\"type\":\"foundation.gas.gas\"}],\"Top\":[]}"
  PS Constant : fl_lib/Physical Signals/Sources/PS Constant  constant=OxyValve.Pressure_Source
  PS-Simulink Converter : nesl_utility/PS-Simulink Converter  PhysicalDomain=network_engine_domain  SubClassName=ps_output  LeftPortType=input  RightPortType=output  PseudoPeriodic=off  Frequencies=[]  VectorFormat=inherit  Unit=Pa  AffineConversion=off
  Percent to Unit : Gain  Gain=Percent_to_Unit
  Pressure & Temperature Sensor (G) : fl_lib/Gas/Sensors/Pressure & Temperature Sensor (G)  reference=foundation.enum.MeasurementReference.difference  pressure=true  pressure_spec=foundation.enum.PressureMeasementSpec.Absolute  temperature=false
      settings: InternalSimscapePortConfiguration="{\"Bottom\":[],\"Left\":[{\"id\":\"A\",\"label\":\"A\",\"type\":\"foundation.gas.gas\"}],\"Right\":[{\"id\":\"B\",\"label\":\"B\",\"type\":\"foundation.gas.gas\"},{\"id\":\"P\",\"label\":\"P\",\"type\":\"output\"}],\"Top\":[]}"
  Simulink-PS Converter : nesl_utility/Simulink-PS Converter  PhysicalDomain=network_engine_domain  SubClassName=ps_input  LeftPortType=input  RightPortType=output  PseudoPeriodic=off  Frequencies=[]  NoiseDistribution=none  NoiseParameters=[]  Unit=1  AffineConversion=off  FilteringAndDerivatives=provide  SimscapeFilterOrder=1  InputFilterTimeConstant=0.001  UdotUserProvided=0
  Unit Conversion : UnitConversion
  B : PMIOPort  Side=Right
  OxySourcePress : Outport  Unit=hPa
  wires:
  OxyVlave/1 -> Data Type Conversion2/1
  Percent to Unit/1 -> Simulink-PS Converter/1
  Unit Conversion/1 -> Data Type Conversion/1
  PS-Simulink Converter/1 -> Unit Conversion/1
  Data Type Conversion/1 -> OxySourcePress/1
  Data Type Conversion2/1 -> Percent to Unit/1
  connections:
  Pressure & Temperature Sensor (G)/RConn1 -- Controlled Pressure Source (G)/LConn1 -- InletReservoir/LConn1
  Simulink-PS Converter/RConn1 -- Orifice (G)/LConn2
  Controlled Pressure Source (G)/RConn1 -- Orifice (G)/LConn1 -- Pressure & Temperature Sensor (G)/LConn1
  PS Constant/RConn1 -- Controlled Pressure Source (G)/LConn2
  Orifice (G)/RConn1 -- B/RConn1
  Pressure & Temperature Sensor (G)/RConn2 -- PS-Simulink Converter/LConn1

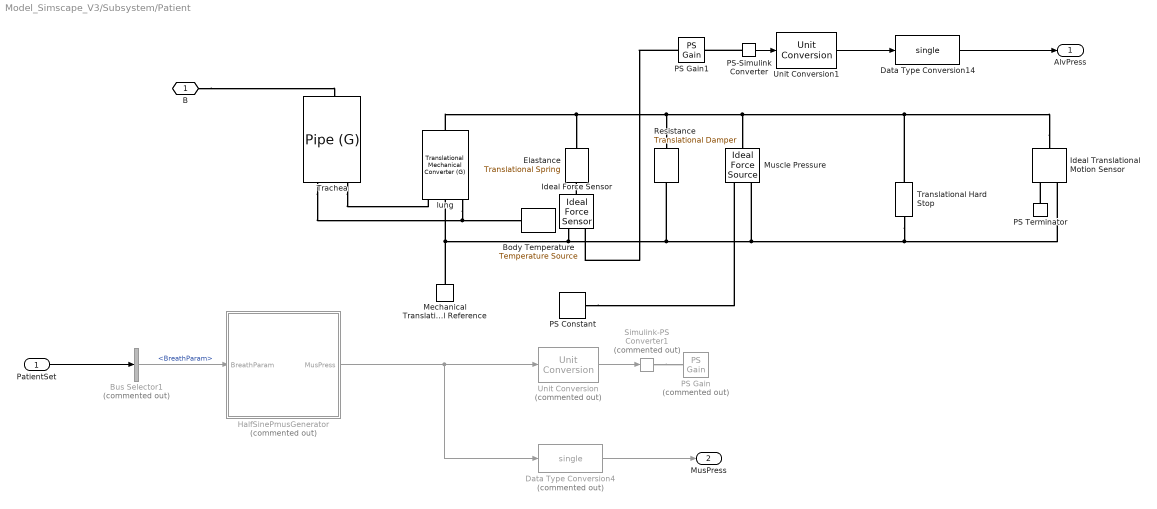
== system Model_Simscape_V3/Subsystem/Patient ==
  PatientSet : Inport
  Body Temperature : fl_lib/Thermal/Thermal Sources/Temperature Source  temperature="Body_Temperature  degC"
  Bus Selector1 : BusSelector  Commented=on  OutputSignals=BreathParam
  Data Type Conversion14 : DataTypeConversion  OutDataTypeStr=single  SaturateOnIntegerOverflow=off  RndMeth=Floor
  Data Type Conversion4 : DataTypeConversion  Commented=on  OutDataTypeStr=single  SaturateOnIntegerOverflow=off  RndMeth=Floor
  Elastance : fl_lib/Mechanical/Translational Elements/Translational Spring  spr_rate=E_respriatory*(lung.Interface_area^2)*(cmH2O_to_Pa/L_to_m3) N/m  v_specify=off  v_priority=None  v=0 m/s  v_nominal_specify=off  v_nominal_unit=m/s  v_nominal_value=1  f_specify=off  f_priority=None  f=0 N  f_nominal_specify=off  f_nominal_unit=N  f_nominal_value=1  x_specify=off  x_priority=High  x=0 m  x_nominal_specify=off  x_nominal_unit=m  x_nominal_value=1
  HalfSinePmusGenerator : Stateflow chart  Commented=on  TreatAsAtomicUnit=on
      settings: AttributesFormatString=半正弦形式等效作用力发生器
  Ideal Force Sensor : fl_lib/Mechanical/Mechanical Sensors/Ideal Force Sensor
  Ideal Translational Motion Sensor : fl_lib/Mechanical/Mechanical Sensors/Ideal Translational Motion Sensor  reference=foundation.enum.MeasurementReference.difference  acceleration_port=false  velocity_port=false  position_port=true  offset=FRC*L_to_m3 m
      settings: InternalSimscapePortConfiguration="{\"Bottom\":[],\"Left\":[{\"id\":\"R\",\"label\":\"R\",\"type\":\"foundation.mechanical.translational.translational\"}],\"Right\":[{\"id\":\"C\",\"label\":\"C\",\"type\":\"foundation.mechanical.translational.translational\"},{\"id\":\"P\",\"label\":\"P\",\"type\":\"output\"}],\"Top\":[]}"
  Mechanical Translational Reference : fl_lib/Mechanical/Translational Elements/Mechanical Translational Reference
  Muscle Pressure : fl_lib/Mechanical/Mechanical Sources/Ideal Force Source
  PS Constant : fl_lib/Physical Signals/Sources/PS Constant  constant=0 N
  PS Gain : fl_lib/Physical Signals/Functions/PS Gain  Commented=on  gain=lung.Interface_area m^2
  PS Gain1 : fl_lib/Physical Signals/Functions/PS Gain  gain=1/lung.Interface_area 1/m^2
  PS Terminator : fl_lib/Physical Signals/Sinks/PS Terminator
  PS-Simulink Converter : nesl_utility/PS-Simulink Converter  PhysicalDomain=network_engine_domain  SubClassName=ps_output  LeftPortType=input  RightPortType=output  PseudoPeriodic=off  Frequencies=[]  VectorFormat=inherit  Unit=Pa  AffineConversion=off
  Resistance : fl_lib/Mechanical/Translational Elements/Translational Damper  D=R_respiratory*(lung.Interface_area^2)*(cmH2O_to_Pa/L_to_m3) N*s/m  v_specify=off  v_priority=None  v=0 m/s  v_nominal_specify=off  v_nominal_unit=m/s  v_nominal_value=1  f_specify=off  f_priority=None  f=0 N  f_nominal_specify=off  f_nominal_unit=N  f_nominal_value=1
  Simulink-PS Converter1 : nesl_utility/Simulink-PS Converter  Commented=on  PhysicalDomain=network_engine_domain  SubClassName=ps_input  LeftPortType=input  RightPortType=output  PseudoPeriodic=off  Frequencies=[]  NoiseDistribution=none  NoiseParameters=[]  Unit=Pa  AffineConversion=off  FilteringAndDerivatives=zero  SimscapeFilterOrder=1  InputFilterTimeConstant=0.001  UdotUserProvided=0
  Trachea : fl_lib/Gas/Elements/Pipe (G)  length=Trachea.Pipe_length m  area=Trachea.area m^2  Dh=Trachea.Hydraulic_diameter m  length_add=0.1 m  roughness=15e-6 m  Re_lam=2000  Re_tur=4000  shape_factor=64  Nu_lam=3.66  p_I_specify=off  p_I_priority=High  p_I=0.101325 MPa  p_I_nominal_specify=off  p_I_nominal_unit=MPa  p_I_nominal_value=1  T_I_specify=on  T_I_priority=High  T_I=37 degC  T_I_nominal_specify=off  T_I_nominal_unit=K  T_I_nominal_value=1  rho_I_specify=off  rho_I_priority=None  rho_I=1.2 kg/m^3  rho_I_nominal_specify=off  rho_I_nominal_unit=kg/m^3  rho_I_nominal_value=1
  Translational Hard Stop : fl_lib/Mechanical/Translational Elements/Translational Hard Stop  upper_bnd=Volume_Max*L_to_m3/lung.Interface_area m  lower_bnd=Hard_Stop.Lower_bound m  model=simscape.enum.hardstop.smooth  stiff_up=1e6 N/m  stiff_low=1e6 N/m  D_up=350 N*s/m  D_low=350 N*s/m  transition=0.01 mm  coeff_rest=0.7  v_tol=0.001 m/s  f_tol=0.001 N  x_specify=off  x_priority=High  x=lung.Initial_displacement m  x_nominal_specify=off  x_nominal_unit=m  x_nominal_value=1  v_specify=off  v_priority=None  v=0 m/s  v_nominal_specify=off  v_nominal_unit=m/s  v_nominal_value=1  f_specify=off  f_priority=None  f=0 N  f_nominal_specify=off  f_nominal_unit=N  f_nominal_value=1  M_specify=off  M_priority=None  M=0
  Unit Conversion : UnitConversion  Commented=on
  Unit Conversion1 : UnitConversion
  lung : fl_lib/Gas/Elements/Translational Mechanical Converter (G)  mech_orientation=foundation.enum.MechOrientationTranslational.Positive  displacement_spec=foundation.enum.DisplacementSpec.Calculate  length_init=FRC*L_to_m3 m  interface_area=lung.Interface_area m^2  dead_volume=lung.Dead_volume m^3  area_A=lung.Cross_area m^2  environment_spec=foundation.enum.pressure_spec.atmospheric  environment_pressure=0.101325 MPa  p_I_specify=off  p_I_priority=High  p_I=0.101325 MPa  p_I_nominal_specify=off  p_I_nominal_unit=MPa  p_I_nominal_value=1  T_I_specify=on  T_I_priority=High  T_I="Body_Temperature  degC"  T_I_nominal_specify=off  T_I_nominal_unit=K  T_I_nominal_value=1  rho_I_specify=off  rho_I_priority=None  rho_I=1.2 kg/m^3  rho_I_nominal_specify=off  rho_I_nominal_unit=kg/m^3  rho_I_nominal_value=1
      settings: LogSimulationData=on  InternalSimscapePortConfiguration="{\"Bottom\":[],\"Left\":[{\"id\":\"A\",\"label\":\"A\",\"type\":\"foundation.gas.gas\"},{\"id\":\"C\",\"label\":\"C\",\"type\":\"foundation.mechanical.translational.translational\"},{\"id\":\"H\",\"label\":\"H\",\"type\":\"foundation.thermal.thermal\"}],\"Right\":[{\"id\":\"R\",\"label\":\"R\",\"type\":\"foundation.mechanical.translational.translational\"}],\"Top\":[]}"
  B : PMIOPort  Side=Left
  AlvPress : Outport  Unit=hPa
  MusPress : Outport  Port=2  Unit=hPa
  wires:
  Unit Conversion/1 -> Simulink-PS Converter1/1
  PS-Simulink Converter/1 -> Unit Conversion1/1
  Unit Conversion1/1 -> Data Type Conversion14/1
  Data Type Conversion14/1 -> AlvPress/1
  HalfSinePmusGenerator/1(MusPress) -> Data Type Conversion4/1, Unit Conversion/1
  Bus Selector1/1 -> HalfSinePmusGenerator/1(BreathParam)  "<BreathParam>"
  PatientSet/1 -> Bus Selector1/1
  Data Type Conversion4/1 -> MusPress/1
  connections:
  Trachea/LConn1 -- lung/LConn1
  Resistance/RConn1 -- Ideal Force Sensor/RConn1 -- Mechanical Translational Reference/LConn1 -- lung/LConn2 -- Translational Hard Stop/RConn1 -- Ideal Translational Motion Sensor/RConn1 -- Muscle Pressure/RConn2
  Ideal Translational Motion Sensor/LConn1 -- lung/RConn1 -- Elastance/LConn1 -- Resistance/LConn1 -- Muscle Pressure/LConn1 -- Translational Hard Stop/LConn1
  PS Terminator/LConn1 -- Ideal Translational Motion Sensor/RConn2
  Trachea/LConn2 -- lung/LConn3 -- Body Temperature/LConn1
  B/RConn1 -- Trachea/RConn1
  Simulink-PS Converter1/RConn1 -- PS Gain/LConn1
  PS Gain1/LConn1 -- Ideal Force Sensor/RConn2
  PS-Simulink Converter/LConn1 -- PS Gain1/RConn1
  PS Constant/RConn1 -- Muscle Pressure/RConn1
  Ideal Force Sensor/LConn1 -- Elastance/RConn1

== system Model_Simscape_V3/Subsystem/TurboFlowSensor ==
  Data Type Conversion5 : DataTypeConversion  OutDataTypeStr=single  SaturateOnIntegerOverflow=off  RndMeth=Floor
  Flow Rate Sensor (G) : fl_lib/Gas/Sensors/Flow Rate Sensor (G)  mass_flow_measure=true  volumetric_flow_measure=true  volumetric_flow_conditions=foundation.enum.volumetric_flow_conditions.actual  p_std=0.101325 MPa  T_std=20 degC  energy_flow_measure=false
      settings: InternalSimscapePortConfiguration="{\"Bottom\":[],\"Left\":[{\"id\":\"A\",\"label\":\"A\",\"type\":\"foundation.gas.gas\"}],\"Right\":[{\"id\":\"B\",\"label\":\"B\",\"type\":\"foundation.gas.gas\"},{\"id\":\"M\",\"label\":\"M\",\"type\":\"output\"},{\"id\":\"V\",\"label\":\"V\",\"type\":\"output\"}],\"Top\":[]}"
  PS Terminator : fl_lib/Physical Signals/Sinks/PS Terminator
  PS-Simulink Converter : nesl_utility/PS-Simulink Converter  PhysicalDomain=network_engine_domain  SubClassName=ps_output  LeftPortType=input  RightPortType=output  PseudoPeriodic=off  Frequencies=[]  VectorFormat=inherit  Unit=m^3/s  AffineConversion=off
  m^3/s to lpm : UnitConversion
  A : PMIOPort  Side=Left
  B : PMIOPort  Port=2  Side=Right
  Flow : Outport  Unit=lpm
  wires:
  m^3/s to lpm/1 -> Data Type Conversion5/1
  PS-Simulink Converter/1 -> m^3/s to lpm/1
  Data Type Conversion5/1 -> Flow/1
  connections:
  Flow Rate Sensor (G)/RConn3 -- PS-Simulink Converter/LConn1
  Flow Rate Sensor (G)/RConn2 -- PS Terminator/LConn1
  Flow Rate Sensor (G)/LConn1 -- A/RConn1
  Flow Rate Sensor (G)/RConn1 -- B/RConn1

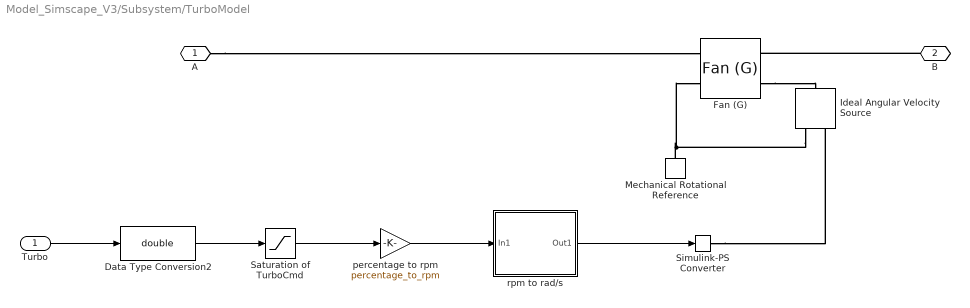
== system Model_Simscape_V3/Subsystem/TurboModel ==
  Turbo : Inport
  Data Type Conversion2 : DataTypeConversion  OutDataTypeStr=double  SaturateOnIntegerOverflow=off  RndMeth=Floor
  Fan (G) : SimscapeFluids_lib/Gas/Turbomachinery/Fan (G)  fan_parameterization=fluids.gas.turbomachinery.enum.FanParameterization.Table2DFlowRate  mechanical_power_spec=fluids.gas.turbomachinery.enum.FanMechanicalPowerSpec.Efficiency  flow_rate_nominal=0.12 m^3/s  pressure_nominal=5400 Pa  eta_nominal=0.40  power_nominal=1620 W  pressure_max=6400 Pa  flow_rate_max=0.24 m^3/s  omega_ref_nominal=3000 rpm  flow_rate_1D_TLU=[.0278, .0556, .0833, .111, .139, .167] m^3/s  pressure_1D_TLU=[6410, 6375, 6018, 5366, 4501, 3609] Pa  eta_1D_TLU=[.257, .394, .453, .47, .459, .415]  power_1D_TLU=[693, 900, 1107, 1267, 1363, 1452] W  omega_ref_1D=3000 rpm  rho_ref_1D=1.2 kg/m^3  omega_threshold_factor=1e-2  omega_dp_TLU=[2400; 3000; 3600] rpm  flow_rate_dp_TLU=[.0278, .0556, .0833, .111, .139, .167] m^3/s  pressure_dp_TLU=[4111, 4010, 3551, 2881, 2167, 1453; 6410, 6375, 6018, 5366, 4501, 3609; 9217, 9285, 9022, 8428, 7552, 6482] Pa  eta_dp_TLU=[.3, .434, .468, .459, .4, .3; .257, .394, .453, .47, .459, .415; .225, .359, .434, .461, .47, .459]  power_dp_TLU=[381, 514, 632, 697, 753, 809; 693, 900, 1107, 1267, 1363, 1452; 1139, 1438, 1732, 2029, 2233, 2358] W  rho_ref_dp=1.2 kg/m^3  omega_q_TLU=Fan.shaftspeed rpm  pressure_q_TLU=Fan.presstable kPa  flow_rate_q_TLU=Fan.flowvector lpm  eta_q_TLU=Fan.efficiency  power_q_TLU=[283, 290, 297, 290; 427, 437, 445, 452; 595, 606, 625, 631] W  rho_ref_q=1.2 kg/m^3  diameter_ratio=1  mech_orientation=fluids.gas.turbomachinery.enum.FanMechanicalOrientation.Positive  area_A=Fan.Inlerarea_A m^2  area_B=Fan.Inlerarea_B m^2
      settings: InternalSimscapePortConfiguration="{\"Bottom\":[],\"Left\":[{\"id\":\"A\",\"label\":\"A\",\"type\":\"foundation.gas.gas\"},{\"id\":\"C\",\"label\":\"C\",\"type\":\"foundation.mechanical.rotational.rotational\"}],\"Right\":[{\"id\":\"B\",\"label\":\"B\",\"type\":\"foundation.gas.gas\"},{\"id\":\"R\",\"label\":\"R\",\"type\":\"foundation.mechanical.rotational.rotational\"}],\"Top\":[]}"
  Ideal Angular Velocity Source : fl_lib/Mechanical/Mechanical Sources/Ideal Angular Velocity Source
  Mechanical Rotational Reference : fl_lib/Mechanical/Rotational Elements/Mechanical Rotational Reference
  Saturation of TurboCmd : Saturate  UpperLimit=CtrlData_Max  LowerLimit=CtrlData_Min
  Simulink-PS Converter : nesl_utility/Simulink-PS Converter  PhysicalDomain=network_engine_domain  SubClassName=ps_input  LeftPortType=input  RightPortType=output  PseudoPeriodic=off  Frequencies=[]  NoiseDistribution=none  NoiseParameters=[]  Unit=rad/s  AffineConversion=off  FilteringAndDerivatives=provide  SimscapeFilterOrder=1  InputFilterTimeConstant=0.001  UdotUserProvided=0
  percentage to rpm : Gain  Gain=percentage_to_rpm
  rpm to rad/s : Subsystem
  A : PMIOPort  Side=Left
  B : PMIOPort  Port=2  Side=Right
  wires:
  rpm to rad/s/1(Out1) -> Simulink-PS Converter/1
  percentage to rpm/1 -> rpm to rad/s/1(In1)
  Turbo/1 -> Data Type Conversion2/1
  Saturation of TurboCmd/1 -> percentage to rpm/1
  Data Type Conversion2/1 -> Saturation of TurboCmd/1
  connections:
  A/RConn1 -- Fan (G)/LConn1
  Ideal Angular Velocity Source/RConn2 -- Mechanical Rotational Reference/LConn1 -- Fan (G)/LConn2
  Fan (G)/RConn2 -- Ideal Angular Velocity Source/LConn1
  Simulink-PS Converter/RConn1 -- Ideal Angular Velocity Source/RConn1
  B/RConn1 -- Fan (G)/RConn1

== system Model_Simscape_V3/Subsystem/ExpValveModel/ Inlet Pressure Sensor ==
  Pressure & Temperature Sensor (G) : fl_lib/Gas/Sensors/Pressure & Temperature Sensor (G)  reference=foundation.enum.MeasurementReference.difference  pressure=true  pressure_spec=foundation.enum.PressureMeasementSpec.Absolute  temperature=false
      settings: InternalSimscapePortConfiguration="{\"Bottom\":[],\"Left\":[{\"id\":\"A\",\"label\":\"A\",\"type\":\"foundation.gas.gas\"}],\"Right\":[{\"id\":\"B\",\"label\":\"B\",\"type\":\"foundation.gas.gas\"},{\"id\":\"P\",\"label\":\"P\",\"type\":\"output\"}],\"Top\":[]}"
  Reservoir (G)1 : fl_lib/Gas/Elements/Reservoir (G)  pressure_spec=foundation.enum.pressure_spec.atmospheric  reservoir_pressure=0.101325 MPa  reservoir_temperature=293.15 K  area_A=Reservoir.Cross_area m^2
  A : PMIOPort  Side=Left
  InletPress : PMIOPort  Port=2  Side=Right
  connections:
  Reservoir (G)1/LConn1 -- Pressure & Temperature Sensor (G)/RConn1
  Pressure & Temperature Sensor (G)/RConn2 -- InletPress/RConn1
  Pressure & Temperature Sensor (G)/LConn1 -- A/RConn1

== system Model_Simscape_V3/Subsystem/ExpValveModel/ Outlet Pressure Sensor ==
  Pressure & Temperature Sensor (G) : fl_lib/Gas/Sensors/Pressure & Temperature Sensor (G)  reference=foundation.enum.MeasurementReference.difference  pressure=true  pressure_spec=foundation.enum.PressureMeasementSpec.Absolute  temperature=false
      settings: InternalSimscapePortConfiguration="{\"Bottom\":[],\"Left\":[{\"id\":\"A\",\"label\":\"A\",\"type\":\"foundation.gas.gas\"}],\"Right\":[{\"id\":\"B\",\"label\":\"B\",\"type\":\"foundation.gas.gas\"},{\"id\":\"P\",\"label\":\"P\",\"type\":\"output\"}],\"Top\":[]}"
  Reservoir (G)1 : fl_lib/Gas/Elements/Reservoir (G)  pressure_spec=foundation.enum.pressure_spec.atmospheric  reservoir_pressure=0.101325 MPa  reservoir_temperature=293.15 K  area_A=Reservoir.Cross_area m^2
  OutletPress : PMIOPort  Side=Left
  A : PMIOPort  Port=2  Side=Right
  connections:
  Pressure & Temperature Sensor (G)/LConn1 -- A/RConn1
  Reservoir (G)1/LConn1 -- Pressure & Temperature Sensor (G)/RConn1
  OutletPress/RConn1 -- Pressure & Temperature Sensor (G)/RConn2

== system Model_Simscape_V3/Subsystem/InspValveModel/ Inlet Pressure Sensor ==
  Pressure & Temperature Sensor (G) : fl_lib/Gas/Sensors/Pressure & Temperature Sensor (G)  reference=foundation.enum.MeasurementReference.difference  pressure=true  pressure_spec=foundation.enum.PressureMeasementSpec.Absolute  temperature=false
      settings: InternalSimscapePortConfiguration="{\"Bottom\":[],\"Left\":[{\"id\":\"A\",\"label\":\"A\",\"type\":\"foundation.gas.gas\"}],\"Right\":[{\"id\":\"B\",\"label\":\"B\",\"type\":\"foundation.gas.gas\"},{\"id\":\"P\",\"label\":\"P\",\"type\":\"output\"}],\"Top\":[]}"
  Reservoir (G)1 : fl_lib/Gas/Elements/Reservoir (G)  pressure_spec=foundation.enum.pressure_spec.atmospheric  reservoir_pressure=0.101325 MPa  reservoir_temperature=293.15 K  area_A=Reservoir.Cross_area m^2
  A : PMIOPort  Side=Left
  InletPress : PMIOPort  Port=2  Side=Right
  connections:
  Reservoir (G)1/LConn1 -- Pressure & Temperature Sensor (G)/RConn1
  Pressure & Temperature Sensor (G)/RConn2 -- InletPress/RConn1
  Pressure & Temperature Sensor (G)/LConn1 -- A/RConn1

== system Model_Simscape_V3/Subsystem/InspValveModel/ Outlet Pressure Sensor ==
  Pressure & Temperature Sensor (G) : fl_lib/Gas/Sensors/Pressure & Temperature Sensor (G)  reference=foundation.enum.MeasurementReference.difference  pressure=true  pressure_spec=foundation.enum.PressureMeasementSpec.Absolute  temperature=false
      settings: InternalSimscapePortConfiguration="{\"Bottom\":[],\"Left\":[{\"id\":\"A\",\"label\":\"A\",\"type\":\"foundation.gas.gas\"}],\"Right\":[{\"id\":\"B\",\"label\":\"B\",\"type\":\"foundation.gas.gas\"},{\"id\":\"P\",\"label\":\"P\",\"type\":\"output\"}],\"Top\":[]}"
  Reservoir (G)1 : fl_lib/Gas/Elements/Reservoir (G)  pressure_spec=foundation.enum.pressure_spec.atmospheric  reservoir_pressure=0.101325 MPa  reservoir_temperature=293.15 K  area_A=Reservoir.Cross_area m^2
  OutletPress : PMIOPort  Side=Left
  A : PMIOPort  Port=2  Side=Right
  connections:
  Pressure & Temperature Sensor (G)/LConn1 -- A/RConn1
  Pressure & Temperature Sensor (G)/RConn2 -- OutletPress/RConn1
  Reservoir (G)1/LConn1 -- Pressure & Temperature Sensor (G)/RConn1

== system Model_Simscape_V3/Subsystem/TurboModel/rpm to rad//s ==
  In1 : Inport  Unit=rpm
  Unit Conversion : UnitConversion
  Out1 : Outport  Unit=rad/s
  wires:
  Unit Conversion/1 -> Out1/1
  In1/1 -> Unit Conversion/1
